simulink model "CVS_LVAD_2021a"  (R2021a)
settings: Solver=ode4  StartTime=0.0  StopTime=end_t  FixedStep=dt_step  RelTol=1e-3
values from neighbouring files (symbols this model uses):
  Cac = 13.7054    [SimMDL_Parameters.m]
  Cbc = 0.25    [SimMDL_Parameters.m]
  Cpa = 1/1.27    (= 0.787401574803)    [SimMDL_Parameters.m]
  Cpv = 1/0.247    (= 4.04858299595)    [SimMDL_Parameters.m]
  Csae = 1/3.02    (= 0.331125827815)    [SimMDL_Parameters.m]
  Csai = 1/7.76    (= 0.128865979381)    [SimMDL_Parameters.m]
  Csve = 1/0.0918    (= 10.8932461874)    [SimMDL_Parameters.m]
  Csvi = 1/0.0989    (= 10.111223458)    [SimMDL_Parameters.m]
  Da0 = 0    [SimMDL_Parameters.m]
  de_gain = 1.5    [SimMDL_Parameters.m]
  delay = 0.5*Tc    (= 0.230769230769)    [SimMDL_Parameters.m]
  deltastar = 0.5    [SimMDL_Parameters.m]
  DElv = 2*(Tc/0.833)    (= 1.10813556192)    [SimMDL_Parameters.m]
  DErv = 2*(Tc/0.833)    (= 1.10813556192)    [SimMDL_Parameters.m]
  Dm0 = 1    [SimMDL_Parameters.m]
  Dp0 = 0    [SimMDL_Parameters.m]
  DRsp = 3*(Tc/0.833)    (= 1.66220334288)    [SimMDL_Parameters.m]
  Dt0 = 1    [SimMDL_Parameters.m]
  dt_step = 1e-3    (= 0.001)    [SimMDL_Parameters.m]
  DTs = 3*(Tc/0.833)    (= 1.66220334288)    [SimMDL_Parameters.m]
  DTv = 0.5    [SimMDL_Parameters.m]
  e_gain = 2    [SimMDL_Parameters.m]
  Elamax = 1.99    [SimMDL_Parameters.m]
  Elamin = 0.733    [SimMDL_Parameters.m]
  Elvmax = 28.4    [SimMDL_Parameters.m]
  Elvmin = 0.550    (= 0.55)    [SimMDL_Parameters.m]
  Eramax = 0.63    [SimMDL_Parameters.m]
  Eramin = 0.317    [SimMDL_Parameters.m]
  Erv_max_sat = 1.2*Ervmax    (= 2.508)    [SimMDL_Parameters.m]
  Erv_max_thres = 0.8*Ervmax    (= 1.672)    [SimMDL_Parameters.m]
  Ervmax = 2.09    [SimMDL_Parameters.m]
  Ervmin = 0.348    [SimMDL_Parameters.m]
  Ga_Elv = 0.012    [SimMDL_Parameters.m]
  Ga_Erv = 0.012    [SimMDL_Parameters.m]
  Ga_Rsp = 0.1    [SimMDL_Parameters.m]
  GaTs = 0.015    [SimMDL_Parameters.m]
  GaTv = 0.028    [SimMDL_Parameters.m]
  Gp_Elv = 0    [SimMDL_Parameters.m]
  Gp_Erv = 0    [SimMDL_Parameters.m]
  Gp_Rsp = 0.33    [SimMDL_Parameters.m]
  GpTs = 0    [SimMDL_Parameters.m]
  GpTv = 0.25    [SimMDL_Parameters.m]
  k_Elv = (Elv_max_sat-Elv_max_thres)/(4*SElvo)    (= 2.84)    [SimMDL_Parameters.m]
  k_Erv = (Erv_max_sat-Erv_max_thres)/(4*SErvo)    (= 0.209)    [SimMDL_Parameters.m]
  k_Rsp = (Rsp_max-Rsp_min)/(4*SRspo)    (= 0.375)    [SimMDL_Parameters.m]
  Kn = max(Kn)    [SimMDL_Parameters.m]
  kT = (T_max-T_min)/(4*STo)    (= 0.035)    [SimMDL_Parameters.m]
  Li = 0.0402    [SimMDL_Parameters.m]
  Lo = 0.0426    [SimMDL_Parameters.m]
  Lsae = 0.0002    [SimMDL_Parameters.m]
  n = length(T)    [SimMDL_Parameters.m]
  pac0 = 0    [SimMDL_Parameters.m]
  pbc0 = 0    [SimMDL_Parameters.m]
  ppa0 = 8.5    [SimMDL_Parameters.m]
  ppv0 = 8    [SimMDL_Parameters.m]
  psae0 = 70    [SimMDL_Parameters.m]
  psai0 = 75    [SimMDL_Parameters.m]
  Psan = 75    [SimMDL_Parameters.m]
  psve0 = 8.7    [SimMDL_Parameters.m]
  psvi0 = 6    [SimMDL_Parameters.m]
  Pth = -3.25    [SimMDL_Parameters.m]
  qi0 = 0    [SimMDL_Parameters.m]
  qo0 = 0    [SimMDL_Parameters.m]
  qsae0 = 10    [SimMDL_Parameters.m]
  Rac = 0.0025    [SimMDL_Parameters.m]
  Ri = 0.4283    [SimMDL_Parameters.m]
  Rm = 0.006    [SimMDL_Parameters.m]
  Ro = 1.2841    [SimMDL_Parameters.m]
  Rpa = 0.006    [SimMDL_Parameters.m]
  Rpp = 0.220    (= 0.22)    [SimMDL_Parameters.m]
  Rpv = 0.006    [SimMDL_Parameters.m]
  Rsae = 0.120    (= 0.12)    [SimMDL_Parameters.m]
  Rsai = 0.016    [SimMDL_Parameters.m]
  Rsp = 2.00    (= 2)    [SimMDL_Parameters.m]
  Rsp_max = 3    [SimMDL_Parameters.m]
  Rsp_min = 1.5    [SimMDL_Parameters.m]
  Rsve = 0.18    [SimMDL_Parameters.m]
  Rsvi = 0.006    [SimMDL_Parameters.m]
  Rtv = 0.006    [SimMDL_Parameters.m]
  t_eject = (Tc*ts_VAD)/dt_step    (= 230.769230769)    [SimMDL_Parameters.m]
  T_max = 0.535    [SimMDL_Parameters.m]
  T_min = 0.395    [SimMDL_Parameters.m]
  Tas = 0.03+0.09*Tc    (= 0.0715384615385)    [SimMDL_Parameters.m]
  Tau_Elv = 1.5    [SimMDL_Parameters.m]
  Tau_Erv = 1.5    [SimMDL_Parameters.m]
  Tau_Rsp = 1.5    [SimMDL_Parameters.m]
  Tau_Ts = 1.8    [SimMDL_Parameters.m]
  Tau_Tv = 0.8    [SimMDL_Parameters.m]
  Tav = 0.01    [SimMDL_Parameters.m]
  Tc = 60/HR    (= 0.461538461538)    [SimMDL_Parameters.m]
  ts_VAD = 0.5    [SimMDL_Parameters.m]
  tune_alpha = x(5)    [SimMDL_Parameters.m]
  tune_gamma = x(3)    [SimMDL_Parameters.m]
  tune_lambda1 = x(1)    [SimMDL_Parameters.m]
  tune_lambda2 = x(2)    [SimMDL_Parameters.m]
  tune_nu = x(4)    [SimMDL_Parameters.m]
  Tvs = 0.16+0.20*Tc    (= 0.252307692308)    [SimMDL_Parameters.m]
  VAD_delay = ts_VAD    (= 0.5)    [SimMDL_Parameters.m]
  vla0 = 11.2524    [SimMDL_Parameters.m]
  Vlau = 1.0    (= 1)    [SimMDL_Parameters.m]
  Vln = 2.3    [SimMDL_Parameters.m]
  vlv0 = 15.6126    [SimMDL_Parameters.m]
  Vlvu = 2.0    (= 2)    [SimMDL_Parameters.m]
  vra0 = 22.36    [SimMDL_Parameters.m]
  Vrau = 1.5    [SimMDL_Parameters.m]
  vrv0 = 26.99    [SimMDL_Parameters.m]
  Vrvu = 3.0    (= 3)    [SimMDL_Parameters.m]
undefined symbols (not defined in the file or in its folder): D_E_max_lv, D_E_max_rv, D_R_svr, D_Ts, D_Tv, f_as_0, f_es_0, f_es_inf, f_es_min, f_ev_0, f_ev_inf, f_max, f_min, G_E_max_lv, G_E_max_rv, G_R_svr, G_Ts, G_Tv, HP_gain, HP_max, HP_min, HP_op, k_es, k_ev, ka, mPsai_op, mPsai_sat, mPsai_thres, passo, pn, Tau_E_max_lv, Tau_E_max_rv, Tau_p, Tau_R_svr, Tau_z
libraries: simulink x6, spsSampleandHoldLib x5, dspmathops x1
(part 1 of 2)
settings Model: SimulationMode=accelerator  Creator=RajarshiB  LastModifiedBy=RajarshiB

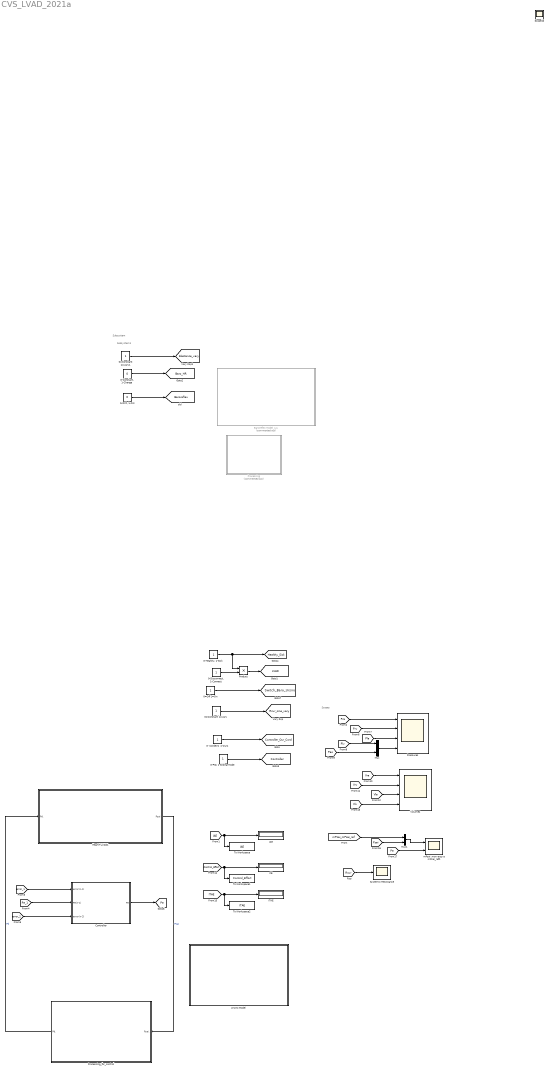
== system CVS_LVAD_2021a ==
  note: Subsystem
  note: Scopes
  note: Subsystem1
  0- Cordeiro  1-Ours : Constant
  "0-Constant, 1-Change" : Constant  Value=0
  "0-Disconnect, 1-Connect" : Constant
  "0-Healthy, 1-Sick" : Constant
  "0-OFF, 1-ON" : Constant  Value=0
  "0-PID, 1-Sliding-Mode" : Constant
  0=Constant 1=vary : Constant
  0=Constant 1=vary1 : Constant
  0=Off 1=On : Constant
  Baroreflex Model_Liu : Subsystem  Commented=on
  CE : Display
  Controller : Subsystem
  Heart+LVAD1 : Subsystem
  IAE : Display
  ITAE : Display
  Mux : Mux  Inputs=2
  Mux1 : Mux  Inputs=2
  Pressures : Scope  NumInputPorts=4
  Processing : Subsystem  Commented=on
  Processing_for_control : Subsystem
  Product : Product
  Systemic Resistance : Scope
  To Workspace : ToWorkspace  VariableName=IAE  SaveFormat=Timeseries  SampleTime=-1
  To Workspace1 : ToWorkspace  VariableName=Control_Effort  SaveFormat=Timeseries  SampleTime=-1
  To Workspace2 : ToWorkspace  VariableName=ITAE  SaveFormat=Timeseries  SampleTime=-1
  Ursino Model : Subsystem
  Volumes : Scope  NumInputPorts=4
  mPsai_mov-avg vs mPsai_ref1 : Scope  NumInputPorts=2
  Scope10 : Scope
  tag scope: Baro_HR=global, Baroreflex=global, Controller=global, Controller_Our_Cord=global, Elastance_vary=global, Healthy_Sick=global, LVAD=global, Pe=global, Rsvr_sine_vary=global, Switch_Baro_Ursino=global
  wires:
  Processing_for_control/1(Pd.) -> Heart+LVAD1/1(Pd.)  "Pd"
  Heart+LVAD1/1(Psai) -> Processing_for_control/1(Psai.)  "Psai"
  Controller/1(Pe) -> [Pe]
  [error_2] -> Controller/3(error(n-2))
  [Pe_1] -> Controller/2(Pe(n-1))
  [error_1] -> Controller/1(error(n-1))
  "0-Disconnect, 1-Connect"/1 -> Product/2
  [IAE] -> To Workspace/1, IAE/1
  "0-PID, 1-Sliding-Mode"/1 -> [Controller]
  "0-Healthy, 1-Sick"/1 -> Product/1, [Healthy_Sick]
  [Pao] -> Mux/2
  [Vrv] -> Volumes/2
  Mux/1 -> Pressures/4
  [Vlv] -> Volumes/4
  [Prv] -> Pressures/2
  [Pla] -> Pressures/3
  [Pra] -> Pressures/1
  [Plv] -> Mux/1
  [Vla] -> Volumes/3
  [Vra] -> Volumes/1
  [mPsai_mPsai_ref] -> Mux1/1
  [Control_Effort] -> To Workspace1/1, CE/1
  [ITAE] -> To Workspace2/1, ITAE/1
  [Psai] -> Mux1/2
  Mux1/1 -> mPsai_mov-avg vs mPsai_ref1/1
  [Pe] -> mPsai_mov-avg vs mPsai_ref1/2
  [Rsvr] -> Systemic Resistance/1
  0=Constant 1=vary/1 -> [Rsvr_sine_vary]
  0=Off 1=On/1 -> [Switch_Baro_Ursino]
  Product/1 -> [LVAD]
  0- Cordeiro  1-Ours/1 -> [Controller_Our_Cord]
  "0-OFF, 1-ON"/1 -> [Baroreflex]
  0=Constant 1=vary1/1 -> [Elastance_vary]
  "0-Constant, 1-Change"/1 -> [Baro_HR]

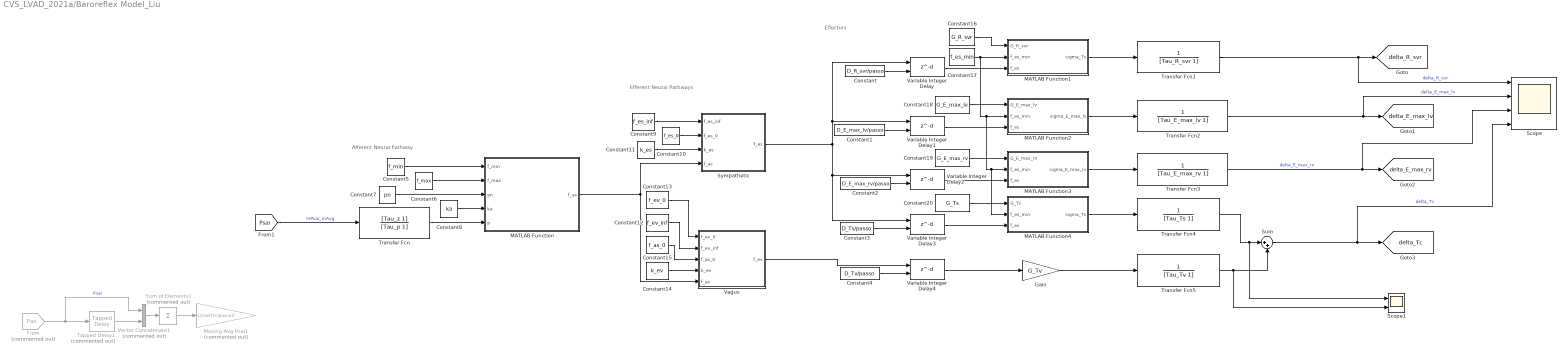
== system CVS_LVAD_2021a/Baroreflex Model_Liu ==
  note: Effectors
  note: Efferent Neural Pathways
  note: Afferent Neural Pathway
  Constant : Constant  Value=D_R_svr/passo
  Constant1 : Constant  Value=D_E_max_lv/passo
  Constant10 : Constant  Value=f_es_0
  Constant11 : Constant  Value=k_es
  Constant12 : Constant  Value=f_ev_inf
  Constant13 : Constant  Value=f_ev_0
  Constant14 : Constant  Value=k_ev
  Constant15 : Constant  Value=f_as_0
  Constant16 : Constant  Value=G_R_svr
  Constant17 : Constant  Value=f_es_min
  Constant18 : Constant  Value=G_E_max_lv
  Constant19 : Constant  Value=G_E_max_rv
  Constant2 : Constant  Value=D_E_max_rv/passo
  Constant20 : Constant  Value=G_Ts
  Constant3 : Constant  Value=D_Ts/passo
  Constant4 : Constant  Value=D_Tv/passo
  Constant5 : Constant  Value=f_min
  Constant6 : Constant  Value=f_max
  Constant7 : Constant  Value=pn
  Constant8 : Constant  Value=ka
  Constant9 : Constant  Value=f_es_inf
  From : From  Commented=on  GotoTag=Pao  TagVisibility=global
  Gain : Gain  Gain=G_Tv
  MATLAB Function : MATLAB Function  TreatAsAtomicUnit=on
  MATLAB Function1 : MATLAB Function  TreatAsAtomicUnit=on
  MATLAB Function2 : MATLAB Function  TreatAsAtomicUnit=on
  MATLAB Function3 : MATLAB Function  TreatAsAtomicUnit=on
  MATLAB Function4 : MATLAB Function  TreatAsAtomicUnit=on
  Moving-Avg Psai1 : Gain  Commented=on  Gain=1/(ceil(Tc/passo))
  Scope : Scope  NumInputPorts=4
  Scope1 : Scope  NumInputPorts=2
  Sum : Sum  Inputs=|++
  Sum of Elements1 : Sum  Commented=on  Inputs=+
  Sympathetic : MATLAB Function  TreatAsAtomicUnit=on
  Tapped Delay1 : simulink/Discrete/Tapped Delay  Commented=on  vinit=psai0  samptime=-1  NumDelays=ceil(Tc/passo)-1  DelayOrder=Oldest  includeCurrent=off
  Transfer Fcn : TransferFcn  Numerator=[Tau_z 1]  Denominator=[Tau_p 1]
  Transfer Fcn1 : TransferFcn  Denominator=[Tau_R_svr 1]
  Transfer Fcn2 : TransferFcn  Denominator=[Tau_E_max_lv 1]
  Transfer Fcn3 : TransferFcn  Denominator=[Tau_E_max_rv 1]
  Transfer Fcn4 : TransferFcn  Denominator=[Tau_Ts 1]
  Transfer Fcn5 : TransferFcn  Denominator=[Tau_Tv 1]
  Vagus : MATLAB Function  TreatAsAtomicUnit=on
  Variable Integer Delay{,1..4} (5 alike) : Delay  DelayLengthSource=Input port
      settings: InputPortMap=u0,p1
  Vector Concatenate1 : Concatenate  Commented=on
  tag scope: delta_E_max_lv=global, delta_E_max_rv=global, delta_R_svr=global, delta_Tc=global
  wires:
  Vagus/1(f_ev) -> Variable Integer Delay4/1
  Constant13/1 -> Vagus/1(f_ev_0)
  MATLAB Function/1(f_as) -> Vagus/5(f_as), Sympathetic/4(f_as)
  Constant18/1 -> MATLAB Function2/1(G_E_max_lv)
  Variable Integer Delay2/1 -> MATLAB Function3/3(f_es)
  Constant17/1 -> MATLAB Function1/2(f_es_min), MATLAB Function2/2(f_es_min), MATLAB Function4/2(f_es_min), MATLAB Function3/2(f_es_min)
  Constant10/1 -> Sympathetic/2(f_es_0)
  Variable Integer Delay3/1 -> MATLAB Function4/3(f_es)
  Constant4/1 -> Variable Integer Delay4/2
  Variable Integer Delay/1 -> MATLAB Function1/3(f_es)
  Transfer Fcn1/1 -> Scope/1, [delta_R_svr]  "delta_R_svr"
  Constant3/1 -> Variable Integer Delay3/2
  Transfer Fcn4/1 -> Scope1/1, Sum/1
  Constant11/1 -> Sympathetic/3(k_es)
  MATLAB Function2/1(sigma_E_max_lv) -> Transfer Fcn2/1
  Sympathetic/1(f_es) -> Variable Integer Delay3/1, Variable Integer Delay2/1, Variable Integer Delay1/1, Variable Integer Delay/1
  Constant5/1 -> MATLAB Function/1(f_min)
  Constant2/1 -> Variable Integer Delay2/2
  Constant12/1 -> Vagus/2(f_ev_inf)
  Variable Integer Delay4/1 -> Gain/1
  MATLAB Function1/1(sigma_Ts) -> Transfer Fcn1/1
  Constant1/1 -> Variable Integer Delay1/2
  Constant14/1 -> Vagus/4(k_ev)
  Constant15/1 -> Vagus/3(f_as_0)
  Constant16/1 -> MATLAB Function1/1(G_R_svr)
  Transfer Fcn/1 -> MATLAB Function/5(p)
  Transfer Fcn3/1 -> Scope/3, [delta_E_max_rv]  "delta_E_max_rv"
  Constant8/1 -> MATLAB Function/4(ka)
  Sum/1 -> Scope/4, [delta_Tc]  "delta_Tc"
  Transfer Fcn2/1 -> Scope/2, [delta_E_max_lv]  "delta_E_max_lv"
  Constant9/1 -> Sympathetic/1(f_es_inf)
  Gain/1 -> Transfer Fcn5/1
  Constant6/1 -> MATLAB Function/2(f_max)
  Constant20/1 -> MATLAB Function4/1(G_Ts)
  Constant/1 -> Variable Integer Delay/2
  Constant7/1 -> MATLAB Function/3(pn)
  Variable Integer Delay1/1 -> MATLAB Function2/3(f_es)
  Transfer Fcn5/1 -> Scope1/2, Sum/2
  MATLAB Function4/1(sigma_Ts) -> Transfer Fcn4/1
  MATLAB Function3/1(sigma_E_max_rv) -> Transfer Fcn3/1
  Constant19/1 -> MATLAB Function3/1(G_E_max_rv)
  Tapped Delay1/1 -> Vector Concatenate1/2
  Vector Concatenate1/1 -> Sum of Elements1/1
  Sum of Elements1/1 -> Moving-Avg Psai1/1
  From/1 -> Vector Concatenate1/1, Tapped Delay1/1  "Psai"
  [Psai] -> Transfer Fcn/1  "mPsai_mAvg"

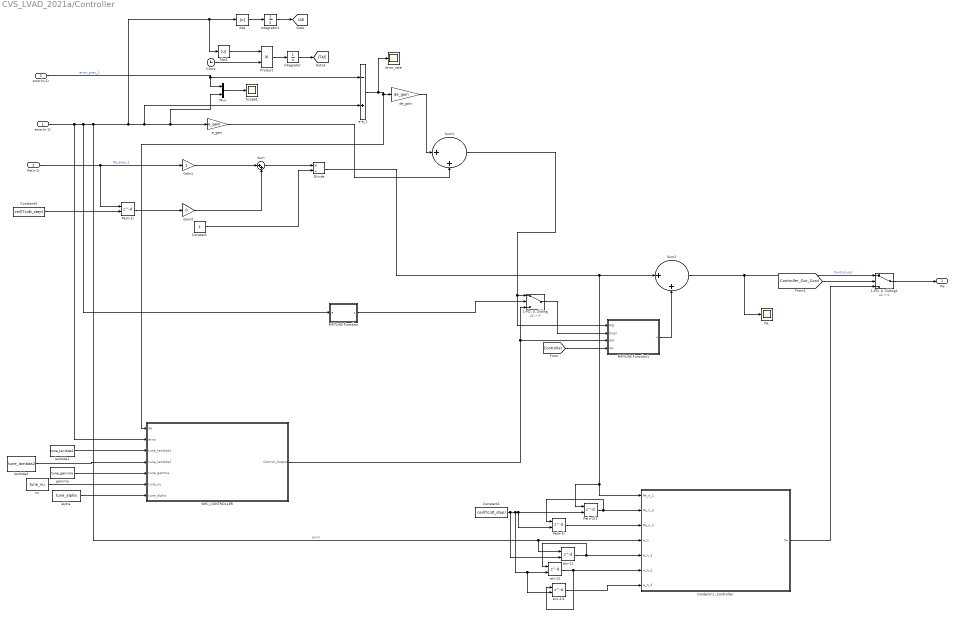
== system CVS_LVAD_2021a/Controller ==
  error(n-1) : Inport
  Pe(n-1) : Inport  Port=2
  error(n-2) : Inport  Port=3
  "1-PD, 0, Sliding" : Switch  Criteria=u2 > Threshold
  "1-PD, 0, Sliding1" : Switch  Criteria=u2 > Threshold
  Abs : Abs
  Abs1 : Abs
  Clock : Clock
  Constant : Constant
  Constant1 : Constant  Value=ceil(Tc/dt_step)
  Constant3 : Constant  Value=ceil(Tc/dt_step)
  Cordeiro's _Controller : MATLAB Function  TreatAsAtomicUnit=on
  Divide : Product  Inputs=*/
  Gain1 : Gain
  Gain3 : Gain  Gain=0
  Integrator : Integrator
  Integrator1 : Integrator
  MATLAB Function : MATLAB Function  TreatAsAtomicUnit=on
  MATLAB Function1 : MATLAB Function  TreatAsAtomicUnit=on
  Mux : Mux  Inputs=2
  Pe(n-2) : Delay  DelayLengthSource=Input port  InitialCondition=120
      settings: InputPortMap=u0,p1
  Pe(n-2)1 : Delay  DelayLengthSource=Input port  InitialCondition=120
      settings: InputPortMap=u0,p1
  Pe(n-3) : Delay  DelayLengthSource=Input port  InitialCondition=120
      settings: InputPortMap=u0,p1
  Pe. : Scope
  Product : Product
  "SMC_CONTROLLER " : Subsystem
  Scope1 : Scope
  Sum : Sum  Inputs=|++
  Sum1 : Sum  Inputs=|++
  Sum2 : Sum  Inputs=|++
  alpha : Constant  Value=tune_alpha
  de_gain : Gain  Gain=de_gain
  e(n-1) : Delay  DelayLengthSource=Input port  InitialCondition=120
      settings: InputPortMap=u0,p1
  e(n-2) : Delay  DelayLengthSource=Input port  InitialCondition=120
      settings: InputPortMap=u0,p1
  e(n-2)1 : Delay  DelayLengthSource=Input port  InitialCondition=120
      settings: InputPortMap=u0,p1
  e-e_1 : Sum  Inputs=-+
  e_gain : Gain  Gain=e_gain
  error_rate : Scope
  gamma : Constant  Value=tune_gamma
  lambda1 : Constant  Value=tune_lambda1
  lambda2 : Constant  Value=tune_lambda2
  nu : Constant  Value=tune_nu
  Pe : Outport
  tag scope: IAE=global, ITAE=global
  wires:
  Pe(n-1)/1 -> Gain1/1, Pe(n-2)/1  "Pe_prev_1"
  Gain1/1 -> Sum/1
  Mux/1 -> Scope1/1
  error(n-2)/1 -> e-e_1/1, Mux/1  "error_prev_1"
  e-e_1/1 -> error_rate/1, "SMC_CONTROLLER "/1(de), de_gain/1
  de_gain/1 -> Sum1/1
  Abs/1 -> Integrator1/1
  Integrator1/1 -> [IAE]
  Pe(n-2)/1 -> Gain3/1
  Gain3/1 -> Sum/2
  Sum/1 -> Divide/1
  Constant/1 -> Divide/2
  e_gain/1 -> Sum1/2
  Divide/1 -> Sum2/1, Pe(n-2)1/1, Cordeiro's _Controller/1(Pe_n_1)
  Constant3/1 -> Pe(n-2)/2
  Sum2/1 -> Pe./1, "1-PD, 0, Sliding1"/1  "Control_out"
  Sum1/1 -> MATLAB Function1/1(PID), "1-PD, 0, Sliding"/1
  "SMC_CONTROLLER "/1(Control_Output) -> "1-PD, 0, Sliding"/3, MATLAB Function1/3(SM)
  MATLAB Function/1(s) -> "1-PD, 0, Sliding"/2
  "1-PD, 0, Sliding"/1 -> MATLAB Function1/2(Dual)
  [Controller] -> MATLAB Function1/4(sw)
  MATLAB Function1/1(u) -> Sum2/2
  Abs1/1 -> Product/1
  Clock/1 -> Product/2
  Product/1 -> Integrator/1
  Integrator/1 -> [ITAE]
  lambda1/1 -> "SMC_CONTROLLER "/3(tune_lambda1)
  lambda2/1 -> "SMC_CONTROLLER "/4(tune_lambda2)
  gamma/1 -> "SMC_CONTROLLER "/5(tune_gamma)
  nu/1 -> "SMC_CONTROLLER "/6(tune_nu)
  alpha/1 -> "SMC_CONTROLLER "/7(tune_alpha)
  Pe(n-2)1/1 -> Pe(n-3)/1, Cordeiro's _Controller/2(Pe_n_2)
  Pe(n-3)/1 -> Cordeiro's _Controller/3(Pe_n_3)
  e(n-1)/1 -> e(n-2)/1, Cordeiro's _Controller/5(e_n_1)
  error(n-1)/1 -> "SMC_CONTROLLER "/2(error), MATLAB Function/1(e), e(n-1)/1, Cordeiro's _Controller/4(e_n), Abs/1, Abs1/1, e-e_1/2, Mux/2, e_gain/1  "error"
  e(n-2)1/1 -> Cordeiro's _Controller/7(e_n_3)
  e(n-2)/1 -> e(n-2)1/1, Cordeiro's _Controller/6(e_n_2)
  Constant1/1 -> e(n-1)/2, e(n-2)1/2, e(n-2)/2, Pe(n-3)/2, Pe(n-2)1/2
  "1-PD, 0, Sliding1"/1 -> Pe/1
  Cordeiro's _Controller/1(Pe) -> "1-PD, 0, Sliding1"/3
  [Controller_Our_Cord] -> "1-PD, 0, Sliding1"/2

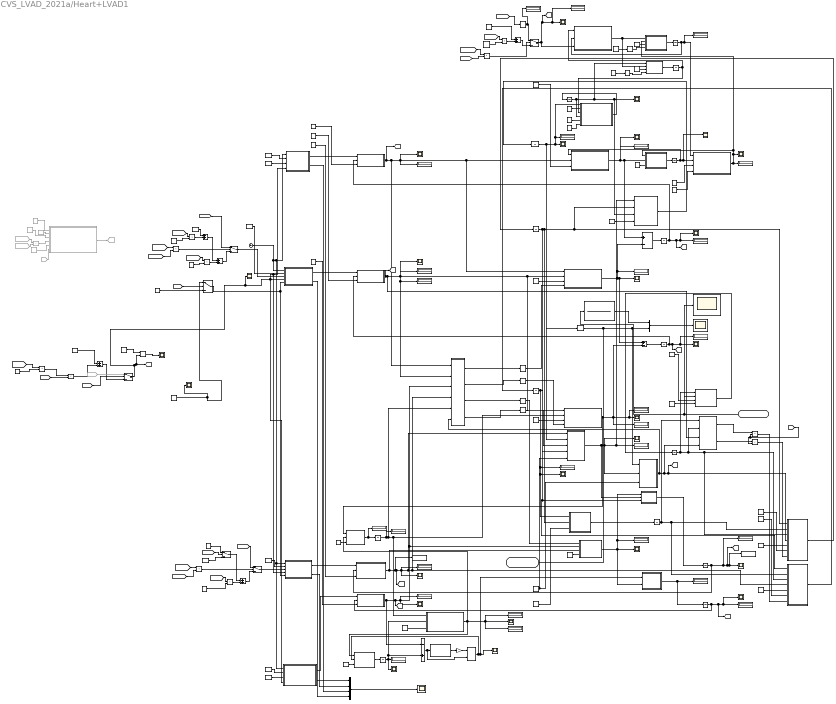
== system CVS_LVAD_2021a/Heart+LVAD1 ==
  note: Subsystem
  note: Subsystem7
  note: qla
  note: Subsystem8
  note: Subsystem1
  note: Subsystem6
  note: Subsystem5
  note: Subsystem3
  note: Subsystem4
  note: Subsystem2
  Pd. : Inport
  Add{,1..4} (5 alike) : Sum
  Clock2 : Clock
  Constant : Constant  Value=Rsai
  Constant1 : Constant  Value=Rsp
  Constant10 : Constant  Value=Cac
  Constant11 : Constant  Value=Ro
  Constant12 : Constant  Value=Lo
  Constant13 : Constant  Value=Csai
  Constant14 : Constant  Value=Csve
  Constant15 : Constant  Value=Csvi
  Constant16 : Constant  Value=Cpa
  Constant17 : Constant  Value=Rsae
  Constant18 : Constant  Value=Lsae
  Constant19 : Constant  Value=Pth
  Constant2 : Constant  Value=Rpa
  Constant20 : Constant  Value=Cpv
  Constant21 : Constant  Value=Rm
  Constant22 : Constant  Value=Kn
  Constant23 : Constant  Commented=on  Value=n
  Constant24 : Constant  Commented=on  Value=Tas
  Constant25 : Constant  Commented=on  Value=Tvs
  Constant26 : Constant  Commented=on  Value=Tav
  Constant27 : Constant  Value=60
  Constant28 : Constant  Value=9
  Constant{29,31,33,35,37} (5 alike) : Constant  Value=0
  Constant3 : Constant  Value=Pth
  Constant30 : Constant  Value=Tc
  Constant36 : Constant  Value=Kn
  Constant4 : Constant  Value=Rpp
  Constant5 : Constant  Value=Rsvi
  Constant6 : Constant  Value=Ri
  Constant7 : Constant  Value=Li
  Constant8 : Constant  Value=Cbc
  Constant9 : Constant  Value=Rac
  Csae : Constant  Value=Csae
  Da0 : Delay  DelayLength=1  InitialCondition=Da0
  Delay : Delay  DelayLength=1  InitialCondition=psai0
  Delay1 : Delay  DelayLength=1  InitialCondition=2
  Derivative : Derivative
  Derivative1 : Derivative
  Display{,1..17} (18 alike) : Display
  Divide : Product  Inputs=*/
  Dm0 : Delay  DelayLength=1  InitialCondition=Dm0
  Dp0 : Delay  DelayLength=1  InitialCondition=Dp0
  Dt0 : Delay  DelayLength=1  InitialCondition=Dt0
  Ela : MATLAB Function  TreatAsAtomicUnit=on
  Elamax : Constant  Value=Elamax
  Elamin : Constant  Value=Elamin
  Elv : MATLAB Function  TreatAsAtomicUnit=on
  Elvmax : Constant  Value=Elvmax
  Elvmin : Constant  Value=Elvmin
  Era : MATLAB Function  TreatAsAtomicUnit=on
  Eramax : Constant  Value=Eramax
  Eramin : Constant  Value=Eramin
  Erv : MATLAB Function  TreatAsAtomicUnit=on
  Ervmax : Constant  Value=Ervmax
  Ervmin : Constant  Value=Ervmin
  From12 : From  Commented=on  GotoTag=iteration  TagVisibility=global
  From21 : From  Commented=on  GotoTag=Baro_Tc
  From8 : From  Commented=on  GotoTag=Baroreflex  TagVisibility=global
  From9 : From  Commented=on  GotoTag=delta_Tc  TagVisibility=global
  Goto : Goto  Commented=on  GotoTag=Kn
  Heart_Valves : MATLAB Function  TreatAsAtomicUnit=on
  Klin : MATLAB Function  TreatAsAtomicUnit=on
  Kn_change : Scope
  Lvad_Valves : MATLAB Function  TreatAsAtomicUnit=on
  MATLAB Function : MATLAB Function  Commented=on  TreatAsAtomicUnit=on
  MiniMod : TransferFcn  Numerator=[1.033 10.74 6.623]  Denominator=[1 6.029 12.98 5.9]  ParameterTunability=Unconstrained
  Mux : Mux
  Mux1 : Mux  Inputs=2
  Pac_ : Integrator  InitialCondition=pac0
  Pao : MATLAB Function  TreatAsAtomicUnit=on
  Pbc_ : Integrator  InitialCondition=pbc0
  Pd : Scope
  Pla : MATLAB Function  TreatAsAtomicUnit=on
  Pla_Scope1 : Scope
  Plv : MATLAB Function  TreatAsAtomicUnit=on
  Plv_Scope2 : Scope
  Ppa : Integrator  InitialCondition=ppa0
  Ppa.. : Display
  Ppv : Integrator  InitialCondition=ppv0
  Ppv_Display : Display
  Pra = Ela*(Vra - Vrau) : MATLAB Function  TreatAsAtomicUnit=on
  Pra_Scope : Scope
  Product{,1..5,7,9..12} (11 alike) : Product
  Product6 : Product  Commented=on
  Prv = Erv*(Vrv - Vrvu) : MATLAB Function  TreatAsAtomicUnit=on
  Prv_Display : Display
  Prv_Scope1 : Scope
  Psae : Integrator  InitialCondition=psae0
  Psai_ : Integrator  InitialCondition=psai0
  Psai_Scope14 : Scope
  Psve : Integrator  InitialCondition=psve0
  Psvi : Integrator  InitialCondition=psvi0
  Rpv_ : Gain  Gain=Rpv
  Rsve : Constant  Value=Rsve
  Rtv : Constant  Value=Rtv
  Scope{,1..16,19} (18 alike) : Scope
  Subtract : Sum  Inputs=-+
  Switch{,1,3..5,7} (6 alike) : Switch  Criteria=u2 > Threshold
  To Workspace : ToWorkspace  VariableName=Plv  SaveFormat=Timeseries  SampleTime=-1
  To Workspace1 : ToWorkspace  VariableName=Vlv  SaveFormat=Timeseries  SampleTime=-1
  Vla : Display
  Vla. : Integrator  InitialCondition=vla0
  Vlau : Constant  Value=Vlau
  Vlv. : Integrator  InitialCondition=vlv0  UpperSaturationLimit=+1000  LowerSaturationLimit=-1000
  Vlvu : Constant  Value=Vlvu
  Vra : Integrator  InitialCondition=vra0
  Vrau : Constant  Value=Vrau
  Vrv : Integrator  InitialCondition=vrv0
  Vrvu : Constant  Value=Vrvu
  Vusae : Constant
  Vusve : Constant
  dPac/dt = (-1/(Rac*Cac))*Pac + (1/(Rac*Cac))*Pd : MATLAB Function  TreatAsAtomicUnit=on
  dPbc/dt = (1/Cbc)*qi - (1/Cbc)*qo : MATLAB Function  TreatAsAtomicUnit=on
  dPpa : Display
  dPpa/dt  = (qpa - qpp)/Cpa : MATLAB Function  TreatAsAtomicUnit=on
  dPpv/dt = (qpp - qla)/Cpv : MATLAB Function  TreatAsAtomicUnit=on
  dPsae/dt  = (qsae - qsp)/Csae : MATLAB Function  TreatAsAtomicUnit=on
  dPsai/dt  = (qsai + qo - qsae)/Csai : MATLAB Function  TreatAsAtomicUnit=on
  dPsve/dt  = (qsp - qsve)/Csve : MATLAB Function  TreatAsAtomicUnit=on
  dPsvi/dt  = (qsve - qra)/Csvi : MATLAB Function  TreatAsAtomicUnit=on
  dVla : Display
  dVla/dt  = qla - qmv : MATLAB Function  TreatAsAtomicUnit=on
  dVlv/dt  = qmv - qsai - qi : MATLAB Function  TreatAsAtomicUnit=on
  dVra/dt  = qra - qtv : Sum  Inputs=+-
  dVrv/dt  = qtv - qpa : Sum  Inputs=+-
  dqi/dt = -(Ri/Li)*qi - Di*(1/Li)*(Pbc+Pac) + Di*(1/Li)*plv : MATLAB Function  TreatAsAtomicUnit=on
  dqo/dt = -(Ro/Lo)*qo + Do*(1/Lo)*(Pac+Pbc) - Do*(1/Lo)*pao : MATLAB Function  TreatAsAtomicUnit=on
  dqsae/dt = (psai + Pth - psae - Rsae*qsae)/Lsae : MATLAB Function  TreatAsAtomicUnit=on
  qi_ : Integrator  InitialCondition=qi0
  qla = (Ppv- Pla)/(klin*Rpv) : Product  Inputs=/*
  qmv : Display
  qmv  = Dm*(Pla -  Plv)/Rmv : MATLAB Function  TreatAsAtomicUnit=on
  qo_ : Integrator  InitialCondition=qo0
  qpa : MATLAB Function  TreatAsAtomicUnit=on
  qpa_Display : Display
  qpp : MATLAB Function  TreatAsAtomicUnit=on
  qpp_Display : Display
  qra : MATLAB Function  TreatAsAtomicUnit=on
  qra_Scope1 : Scope
  qsae_ : Integrator  InitialCondition=qsae0  UpperSaturationLimit=1000  LowerSaturationLimit=-1000
  qsai : MATLAB Function  TreatAsAtomicUnit=on
  qsp : MATLAB Function  TreatAsAtomicUnit=on
  qsve : MATLAB Function  TreatAsAtomicUnit=on
  qtv : MATLAB Function  TreatAsAtomicUnit=on
  qtv_Scope1 : Scope
  qtv_Scope2 : Scope
  Psai : Outport
  tag scope: Pao=global, Pla=global, Plv=global, Pra=global, Prv=global, Rsvr=global, Tc=global, Vla=global, Vlv=global, Vra=global, Vrv=global
  wires:
  MiniMod/1 -> Mux1/1
  Constant11/1 -> dqo/dt = -(Ro/Lo)*qo + Do*(1/Lo)*(Pac+Pbc) - Do*(1/Lo)*pao/5(Ro)
  Constant12/1 -> dqo/dt = -(Ro/Lo)*qo + Do*(1/Lo)*(Pac+Pbc) - Do*(1/Lo)*pao/6(Lo)
  dPac/dt = (-1/(Rac*Cac))*Pac + (1/(Rac*Cac))*Pd/1(dPac) -> Pac_/1
  dqi/dt = -(Ri/Li)*qi - Di*(1/Li)*(Pbc+Pac) + Di*(1/Li)*plv/1(dqi) -> qi_/1
  Vrvu/1 -> Prv = Erv*(Vrv - Vrvu)/3(Vrvu)
  Lvad_Valves/1(Di) -> Product/1
  Constant3/1 -> qsve/3(Pth)
  Heart_Valves/1(Dt) -> Dt0/1
  Constant13/1 -> dPsai/dt  = (qsai + qo - qsae)/Csai/4(Csai)
  Prv = Erv*(Vrv - Vrvu)/1(Prv) -> [Prv], Display1/1, Heart_Valves/2(Prv), qpa/1(Prv), qtv/2(Prv), Prv_Display/1, Prv_Scope1/1, Lvad_Valves/3(Plv)
  Elamin/1 -> Ela/2(Elamin)
  Mux/1 -> Scope2/1
  Era/2(avt) -> Mux/3
  Clock2/1 -> Ela/1(Time), Elv/1(Time), Era/1(Time), Erv/1(Time)
  Constant2/1 -> qpa/3(Rpa)
  dPsve/dt  = (qsp - qsve)/Csve/1(Psve) -> Psve/1
  Product1/1 -> dqo/dt = -(Ro/Lo)*qo + Do*(1/Lo)*(Pac+Pbc) - Do*(1/Lo)*pao/7(Do)
  dPpa/dt  = (qpa - qpp)/Cpa/1(dPpa) -> dPpa/1, Ppa/1
  Vlau/1 -> Pla/3(Vlau)
  Heart_Valves/3(Dm) -> Dm0/1
  Rsve/1 -> qsve/4(Rsve)
  Constant14/1 -> dPsve/dt  = (qsp - qsve)/Csve/3(Csve)
  Eramin/1 -> Era/2(Eramin)
  dqsae/dt = (psai + Pth - psae - Rsae*qsae)/Lsae/1(dqsae) -> qsae_/1
  Elv/2(avt) -> Mux/2
  Constant4/1 -> qpp/3(Rpp)
  Ela/1(Ela) -> Pla/1(Ela)
  Erv/1(Erv) -> Prv = Erv*(Vrv - Vrvu)/1(Erv)
  Rtv/1 -> qtv/3(Rtv)
  Heart_Valves/2(Dp) -> Dp0/1
  dPpv/dt = (qpp - qla)/Cpv/1(dPpv) -> Ppv/1
  Heart_Valves/4(Da) -> Da0/1
  Eramax/1 -> Era/3(Eramax)
  Lvad_Valves/2(Do) -> Product1/1
  Dp0/1 -> qpa/4(Dp)
  Ervmin/1 -> Erv/2(Ervmin)
  Delay/1 -> Mux1/2, Pao/1(Psai), Psai/1
  Constant9/1 -> dPac/dt = (-1/(Rac*Cac))*Pac + (1/(Rac*Cac))*Pd/3(Rac)
  Product/1 -> dqi/dt = -(Ri/Li)*qi - Di*(1/Li)*(Pbc+Pac) + Di*(1/Li)*plv/7(Di)
  Vlvu/1 -> Plv/3(Vlvu)
  Pd./1 -> dPac/dt = (-1/(Rac*Cac))*Pac + (1/(Rac*Cac))*Pd/2(Pd), MiniMod/1, Pd/1  "Pd"
  Elvmin/1 -> Elv/2(Elvmin)
  Vrau/1 -> Pra = Ela*(Vra - Vrau)/3(Vrau)
  Subtract/1 -> Klin/1(Ppv_Pla), qla = (Ppv- Pla)/(klin*Rpv)/2
  dPbc/dt = (1/Cbc)*qi - (1/Cbc)*qo/1(dPbc) -> Pbc_/1
  Switch/1 -> Elv/3(Elvmax)
  dPsai/dt  = (qsai + qo - qsae)/Csai/1(dPsai) -> Psai_/1
  Psae/1 -> dqsae/dt = (psai + Pth - psae - Rsae*qsae)/Lsae/3(Psae), qsp/1(Psae)
  dVlv/dt  = qmv - qsai - qi/1(dVlv) -> Vlv./1
  Dt0/1 -> qtv/4(Dt)
  Constant6/1 -> dqi/dt = -(Ri/Li)*qi - Di*(1/Li)*(Pbc+Pac) + Di*(1/Li)*plv/5(Ri)
  Era/1(Era) -> Pra = Ela*(Vra - Vrau)/1(Era)
  Switch5/1 -> Erv/3(Ervmax)
  Ela/2(avt) -> Mux/1
  Elv/1(Elv) -> Plv/1(Elv)
  Erv/2(avt) -> Mux/4
  Da0/1 -> qsai/3(Da)
  Mux1/1 -> Scope15/1
  qsve/1(qsve) -> dPsve/dt  = (qsp - qsve)/Csve/2(qsve), dPsvi/dt  = (qsve - qra)/Csvi/1(qsve), qtv_Scope2/1, Display6/1  "qsve"
  Switch7/1 -> Elv/4(Tc), Era/4(Tc), Erv/4(Tc), Ela/4(Tc), Scope10/1, Divide/2, [Tc]  "HR"
  Elamax/1 -> Ela/3(Elamax)
  Constant8/1 -> dPbc/dt = (1/Cbc)*qi - (1/Cbc)*qo/3(Cbc)
  Constant7/1 -> dqi/dt = -(Ri/Li)*qi - Di*(1/Li)*(Pbc+Pac) + Di*(1/Li)*plv/6(Li)
  Constant10/1 -> dPac/dt = (-1/(Rac*Cac))*Pac + (1/(Rac*Cac))*Pd/4(Cac)
  dqo/dt = -(Ro/Lo)*qo + Do*(1/Lo)*(Pac+Pbc) - Do*(1/Lo)*pao/1(dqo) -> qo_/1
  Constant5/1 -> qra/3(Rsvi)
  qo_/1 -> dPsai/dt  = (qsai + qo - qsae)/Csai/2(qo), dqo/dt = -(Ro/Lo)*qo + Do*(1/Lo)*(Pac+Pbc) - Do*(1/Lo)*pao/1(qo), dPbc/dt = (1/Cbc)*qi - (1/Cbc)*qo/2(qo), qsai/4(qo)  "qo"
  Pbc_/1 -> dqo/dt = -(Ro/Lo)*qo + Do*(1/Lo)*(Pac+Pbc) - Do*(1/Lo)*pao/2(Pbc), dqi/dt = -(Ri/Li)*qi - Di*(1/Li)*(Pbc+Pac) + Di*(1/Li)*plv/2(Pbc), Lvad_Valves/1(Pbc)
  qtv/1(qtv) -> dVrv/dt  = qtv - qpa/1, qtv_Scope1/1, dVra/dt  = qra - qtv/2, Display5/1  "qtv"
  qsai/1(qsai) -> Display13/1, dPsai/dt  = (qsai + qo - qsae)/Csai/1(qsai), Pao/2(qsai), Scope8/1, dVlv/dt  = qmv - qsai - qi/2(qsai)
  Pao/1(Pao_) -> [Pao], dqo/dt = -(Ro/Lo)*qo + Do*(1/Lo)*(Pac+Pbc) - Do*(1/Lo)*pao/4(Pao), Lvad_Valves/4(Pao), Heart_Valves/6(Pao)
  qi_/1 -> dPbc/dt = (1/Cbc)*qi - (1/Cbc)*qo/1(qi), Scope6/1, Display11/1, dqi/dt = -(Ri/Li)*qi - Di*(1/Li)*(Pbc+Pac) + Di*(1/Li)*plv/1(qi), dVlv/dt  = qmv - qsai - qi/3(qi)
  Constant/1 -> Pao/3(Rsai), qsai/5(Rsai)
  Vlv./1 -> Display10/1, [Vlv], To Workspace1/1, Scope5/1, Plv/2(Vlv)
  Constant15/1 -> dPsvi/dt  = (qsve - qra)/Csvi/3(Csvi)
  Psai_/1 -> dqsae/dt = (psai + Pth - psae - Rsae*qsae)/Lsae/1(Psai), Display14/1, Psai_Scope14/1, qsai/2(Psai), Delay/1  "Psai"
  qsp/1(qsp) -> dPsve/dt  = (qsp - qsve)/Csve/1(qsp), dPsae/dt  = (qsae - qsp)/Csae/2(qsp)  "qsp"
  Vla./1 -> [Vla], Scope13/1, Vla/1, Pla/2(Vla)
  Ppa/1 -> qpp/1(Ppa), qpa/2(Ppa), Heart_Valves/5(Ppa), Ppa../1
  Plv/1(Plv) -> To Workspace/1, [Plv], Heart_Valves/4(Plv), dqi/dt = -(Ri/Li)*qi - Di*(1/Li)*(Pbc+Pac) + Di*(1/Li)*plv/4(Plv), qsai/1(Plv), Plv_Scope2/1, Display2/1, qmv  = Dm*(Pla -  Plv)/Rmv/3(Plv)
  Pra = Ela*(Vra - Vrau)/1(Pra) -> [Pra], qtv/1(Pra), qra/2(Pra), Display/1, Pra_Scope/1, Heart_Valves/1(Pra)
  dVla/dt  = qla - qmv/1(dVla) -> dVla/1, Vla./1
  [LVAD] -> Product/2, Product1/2
  qra/1(qra) -> dVra/dt  = qra - qtv/1, dPsvi/dt  = (qsve - qra)/Csvi/2(qra), Display4/1, qra_Scope1/1
  Pla/1(Pla) -> [Pla], qmv  = Dm*(Pla -  Plv)/Rmv/2(Pla), Heart_Valves/3(Pla), Pla_Scope1/1, Display3/1, Subtract/1
  Switch3/1 -> [Rsvr], Display15/1, Scope14/1, qsp/3(Rsp)
  Pac_/1 -> dqo/dt = -(Ro/Lo)*qo + Do*(1/Lo)*(Pac+Pbc) - Do*(1/Lo)*pao/3(Pac), dqi/dt = -(Ri/Li)*qi - Di*(1/Li)*(Pbc+Pac) + Di*(1/Li)*plv/3(Pac), Lvad_Valves/2(Pac), dPac/dt = (-1/(Rac*Cac))*Pac + (1/(Rac*Cac))*Pd/1(Pac)
  qpa/1(qpa) -> Scope1/1, Display8/1, dVrv/dt  = qtv - qpa/2, qpa_Display/1, dPpa/dt  = (qpa - qpp)/Cpa/1(qpa)
  Vrv/1 -> [Vrv], Display9/1, Scope4/1, Prv = Erv*(Vrv - Vrvu)/2(Vrv)
  qpp/1(qpp) -> qpp_Display/1, Display12/1, Scope7/1, dPpv/dt = (qpp - qla)/Cpv/1(qpp), dPpa/dt  = (qpa - qpp)/Cpa/2(qpp)
  Constant16/1 -> dPpa/dt  = (qpa - qpp)/Cpa/3(Cpa)
  Constant20/1 -> dPpv/dt = (qpp - qla)/Cpv/3(Cpv)
  Ppv/1 -> Subtract/2, qpp/2(Ppv), Ppv_Display/1, Scope11/1
  Constant21/1 -> qmv  = Dm*(Pla -  Plv)/Rmv/4(Rmv)
  qmv  = Dm*(Pla -  Plv)/Rmv/1(qmv) -> dVlv/dt  = qmv - qsai - qi/1(qmv), qmv/1, Scope9/1, dVla/dt  = qla - qmv/2(qmv)
  dPsvi/dt  = (qsve - qra)/Csvi/1(dPsvi) -> Psvi/1
  Psvi/1 -> Scope16/1, qsve/2(Psvi), qra/1(Psvi)
  Klin/1(Klin) -> Rpv_/1
  Rpv_/1 -> qla = (Ppv- Pla)/(klin*Rpv)/1
  qla = (Ppv- Pla)/(klin*Rpv)/1 -> dVla/dt  = qla - qmv/1(qla), Scope12/1, dPpv/dt = (qpp - qla)/Cpv/2(qla)
  Psve/1 -> Display16/1, qsve/1(Psve), qsp/2(Psve)
  Csae/1 -> dPsae/dt  = (qsae - qsp)/Csae/3(Csae)
  dPsae/dt  = (qsae - qsp)/Csae/1(dPsae) -> Psae/1
  Constant17/1 -> dqsae/dt = (psai + Pth - psae - Rsae*qsae)/Lsae/5(Rsae)
  Constant19/1 -> dqsae/dt = (psai + Pth - psae - Rsae*qsae)/Lsae/2(Pth)
  Constant18/1 -> dqsae/dt = (psai + Pth - psae - Rsae*qsae)/Lsae/6(Lsae)
  qsae_/1 -> dPsai/dt  = (qsai + qo - qsae)/Csai/3(qsae), Scope/1, dPsae/dt  = (qsae - qsp)/Csae/1(qsae), dqsae/dt = (psai + Pth - psae - Rsae*qsae)/Lsae/4(qsae)  "qsae"
  dVrv/dt  = qtv - qpa/1 -> Vrv/1
  dVra/dt  = qra - qtv/1 -> Vra/1
  Vra/1 -> [Vra], Scope3/1, Display7/1, Pra = Ela*(Vra - Vrau)/2(Vra)  "Vra"
  Dm0/1 -> qmv  = Dm*(Pla -  Plv)/Rmv/1(Dm)
  [Baroreflex] -> Product2/1
  Constant29/1 -> Product2/2
  Product2/1 -> Add/2
  Ervmax/1 -> Add/1
  Product3/1 -> Add1/2
  Switch1/1 -> Add1/1
  Constant33/1 -> Product3/2
  [Baroreflex] -> Product3/1
  Product4/1 -> Add2/2
  Constant1/1 -> Add2/1
  Constant37/1 -> Product4/2
  [Baroreflex] -> Product4/1
  MATLAB Function/1(Kn) -> Goto/1
  From9/1 -> Product6/2
  From8/1 -> Product6/1
  Product6/1 -> MATLAB Function/4(Tc)
  Constant23/1 -> MATLAB Function/5(n)
  Constant24/1 -> MATLAB Function/1(Tas)
  Constant26/1 -> MATLAB Function/2(Tav)
  Constant25/1 -> MATLAB Function/3(Tvs)
  From12/1 -> MATLAB Function/6(iter)
  Constant28/1 -> Switch1/1
  [Healthy_Sick] -> Switch1/2
  Elvmax/1 -> Switch1/3
  Add4/1 -> Switch7/3  "Tc"
  [Baroreflex] -> Product9/1
  Constant31/1 -> Product9/2
  Constant30/1 -> Add4/1  "Tc0"
  Product9/1 -> Product5/1
  [Baro_HR] -> Switch4/2
  Constant36/1 -> Kn_change/1, Switch4/1  "Kn"
  Constant22/1 -> Switch4/3
  Switch4/1 -> Erv/5(Kn), Elv/5(Kn)  "Kn"
  From21/1 -> Switch7/1
  [Baro_HR] -> Switch7/2
  [Baro_HR] -> Product5/2
  Product5/1 -> Add4/2
  Constant27/1 -> Divide/1
  Divide/1 -> Scope19/1  "HR"
  Add2/1 -> Switch3/3
  Delay1/1 -> Display17/1, Switch3/1
  Product7/1 -> Switch3/2
  [Baro_Rsp] -> Delay1/1
  [Switch_Baro_Ursino] -> Product7/1
  [Rsvr_sine_vary] -> Product7/2
  Vusae/1 -> Derivative/1
  Derivative/1 -> dPsae/dt  = (qsae - qsp)/Csae/4(Vusae_dot)
  Vusve/1 -> Derivative1/1
  Derivative1/1 -> dPsve/dt  = (qsp - qsve)/Csve/4(Vusve_dot)
  Add1/1 -> Switch/3
  [Switch_Baro_Ursino] -> Product10/1
  [Elastance_vary] -> Product10/2
  Product10/1 -> Switch/2
  [Elv_baro_ursino] -> Switch/1
  Product11/1 -> Switch5/2
  Add3/1 -> Switch5/3
  Product12/1 -> Add3/2
  [Baroreflex] -> Product12/1
  Add/1 -> Add3/1
  Constant35/1 -> Product12/2
  [Elastance_vary] -> Product11/2
  [Switch_Baro_Ursino] -> Product11/1
  [Erv_baro_ursino] -> Switch5/1

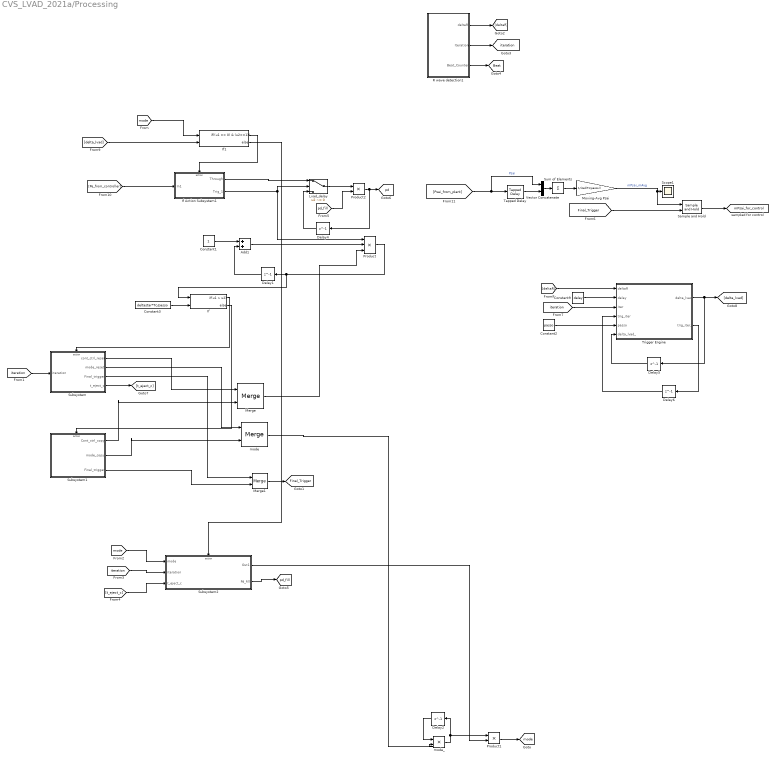
== system CVS_LVAD_2021a/Processing ==
  Add1 : Sum
  Constant1 : Constant
  Constant2 : Constant  Value=passo
  Constant3 : Constant  Value=deltastar*Tc/passo
  Constant9 : Constant  Value=delay
  Delay{1,4..6} (4 alike) : Delay  DelayLength=1
  Delay2 : Delay  DelayLength=1  InitialCondition=0
  If : If  NumInputs=2  IfExpression=u1 > u2
  If Action Subsystem1 : Subsystem  TreatAsAtomicUnit=on
  If1 : If  NumInputs=2  IfExpression=(u1 == 0) & (u2==1)
  Lvad_delay : Switch  Criteria=u2 ~= 0
  Merge : Merge
  Merge1 : Merge
  Moving-Avg Psai : Gain  Gain=1/(ceil(Tc/passo))
  Product : Product  Inputs=3
  Product1 : Product
  Product2 : Product
  R wave detection1 : Subsystem
  Sample and Hold : spsSampleandHoldLib/Sample and Hold  ic=0  Ts=passo
      settings: SourceProductBaseCode=PS
  Scope1 : Scope
  Subsystem : Subsystem
  Subsystem1 : Subsystem
  Subsystem2 : Subsystem
  Sum of Elements : Sum  Inputs=+
  Tapped Delay : simulink/Discrete/Tapped Delay  vinit=psai0  samptime=-1  NumDelays=ceil(Tc/passo)-1  DelayOrder=Oldest  includeCurrent=off
  Trigger Engine : MATLAB Function  TreatAsAtomicUnit=on
  Vector Concatenate : Concatenate
  mode : Merge
  mode_ : Product
  tag scope: Beat=global, Final_Trigger=global, iteration=global, mPsai_for_control=global, mode=global, pd=global, pd_fill=global
  wires:
  Sum of Elements/1 -> Moving-Avg Psai/1
  Constant9/1 -> Trigger Engine/2(delay)
  Lvad_delay/1 -> Product2/1
  [Psai_from_plant] -> Vector Concatenate/1, Tapped Delay/1  "Psai"
  Tapped Delay/1 -> Vector Concatenate/2
  Sample and Hold/1 -> [mPsai_for_control]
  Product/1 -> If/1, Delay1/1
  If Action Subsystem1/1(Through) -> Lvad_delay/1
  If/1 -> Subsystem/Action
  Trigger Engine/2(trig_iter_) -> Delay6/1
  Product2/1 -> Delay4/1, [pd]
  Product1/1 -> [mode]
  [Final_Trigger] -> Sample and Hold/2
  Add1/1 -> Product/2
  mode_/1 -> Delay2/1, Product1/1
  Vector Concatenate/1 -> Sum of Elements/1
  Constant2/1 -> Trigger Engine/5(passo)
  Delay1/1 -> Add1/2
  Trigger Engine/1(delta_lvad) -> Delay5/1, [delta_lvad]
  Moving-Avg Psai/1 -> Sample and Hold/1, Scope1/1  "mPsai_mAvg"
  Delay4/1 -> Lvad_delay/3
  If1/1 -> If Action Subsystem1/Action
  Delay2/1 -> mode_/1
  R wave detection1/3(Beat_Counter) -> [Beat]
  [Pe_from_controller] -> If Action Subsystem1/1(In1)
  [mode] -> If1/1
  Delay6/1 -> Trigger Engine/4(trig_iter)
  [delta_lvad] -> If1/2
  mode/1 -> mode_/2
  Constant3/1 -> If/2
  R wave detection1/1(deltaR) -> [deltaR]
  R wave detection1/2(Iteration) -> [iteration]
  Merge/1 -> Product/3
  Constant1/1 -> Add1/1
  [deltaR] -> Trigger Engine/1(deltaR)
  [pd_fill] -> Product2/2
  [iteration] -> Trigger Engine/3(iter)
  Delay5/1 -> Trigger Engine/6(delta_lvad_)
  Subsystem/1(cont_ctrl_reset) -> Merge/1
  Subsystem/2(mode_reset) -> mode/1
  Subsystem1/1(Cont_ctrl_copy) -> Merge/2
  Subsystem1/2(mode_copy) -> mode/2
  Subsystem/3(Final_trigger) -> Merge1/1
  Subsystem1/3(Final_trigger) -> Merge1/2
  Merge1/1 -> [Final_Trigger]
  Subsystem/4(t_eject_c) -> [t_eject_c]
  If/2 -> Subsystem1/Action
  [iteration] -> Subsystem/1(iteration)
  If Action Subsystem1/2(Trig_1) -> Product/1, Lvad_delay/2
  Subsystem2/1(Out1) -> Product1/2
  If1/2 -> Subsystem2/Action
  Subsystem2/2(Pd_fill) -> [pd_fill]
  [mode] -> Subsystem2/1(mode)
  [iteration] -> Subsystem2/2(iteration)
  [t_eject_c] -> Subsystem2/3(t_eject_c)

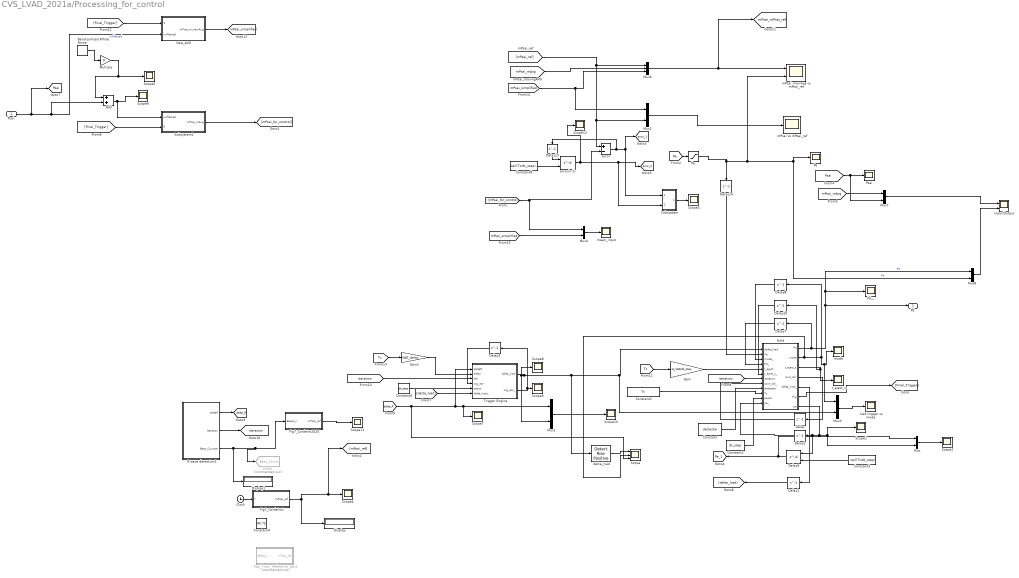
== system CVS_LVAD_2021a/Processing_for_control ==
  Psai. : Inport
  Add : Sum
  Band-Limited White Noise : simulink/Sources/Band-Limited White Noise  Cov=[0.0001]  Ts=dt_step  seed=[23341]
  Clock : Clock
  Constant : Constant  Value=deltastar
  Constant1 : Constant  Value=Tc
  Constant2 : Constant  Value=dt_step
  Constant3 : Constant  Value=ceil(Tc/dt_step)
  Constant4 : Constant  Value=80.75
  Constant6 : Constant  Value=dt_step
  Constant8 : Constant  Value=ceil(Tc/dt_step)-1  SampleTime=-1
  Delay : Delay  DelayLength=1  InitialCondition=0
  Delay1 : Delay  DelayLength=1  InitialCondition=0
  Delay10 : Delay  DelayLength=1  InitialCondition=t_eject
  Delay{3,7,13..14} (4 alike) : Delay  DelayLength=1
  Delay2 : Delay  DelayLength=1  InitialCondition=120
  Delay8 : Delay  DelayLength=1  InitialCondition=0
  Delay9 : Delay  DelayLengthSource=Input port  DelayLength=1  DelayLengthUpperLimit=10000  InitialCondition=120
      settings: InputPortMap=u0,p1
  Display : Display
  Display1 : Display
  Fig7_Cordeiro1 : MATLAB Function  TreatAsAtomicUnit=on
  Fig7_Cordeiro2020 : MATLAB Function  TreatAsAtomicUnit=on
  Gain : Gain  Gain=ts_VAD/dt_step
  Gain1 : Gain  Gain=VAD_delay
  Goto6 : Goto  Commented=on  GotoTag=Beat_Count  TagVisibility=global
  Hold : MATLAB Function  TreatAsAtomicUnit=on
  Input/Output : Scope  NumInputPorts=2
  Multiply : Gain  Gain=0
  Mux{,1..4,7..8} (7 alike) : Mux  Inputs=2
      Mux1 settings: DisplayOption=signals
  Mux6 : Mux  Inputs=3
  New_AVG : Subsystem
  Pd__ : Scope
  Pe : Scope
  Pe. : Saturate  UpperLimit=300  LowerLimit=-20
  Psai : Scope
  Psai_Train_Reference_gen1 : MATLAB Function  Commented=on  TreatAsAtomicUnit=on
  R wave detection1 : Subsystem
  Scope : Scope  NumInputPorts=3
  Scope{1..12} (12 alike) : Scope
  Subsystem : Subsystem
  Subsystem1 : Subsystem
  Trigger Engine : MATLAB Function  TreatAsAtomicUnit=on
  delta_lvad : simulink/Logic and Bit Operations/Detect Rise Positive  vinit=0  OutDataTypeStr=boolean
  error : Sum  Inputs=+-
  error(n-1). : Delay  DelayLengthSource=Input port  DelayLength=1  DelayLengthUpperLimit=10000  InitialCondition=0  SampleTime=dt_step
      settings: InputPortMap=u0,p1
  lvad trigger vs mode : Scope
  mPsai vs mPsai_ref : Scope
  mPsai_mov-avg vs mPsai_ref : Scope  NumInputPorts=2
  mean_input : Scope
  mode : Scope
  t_eject_c : Scope
  Pd. : Outport
  tag scope: Pe_1=global, Psai=global, delta_R=global, error_1=global, error_2=global, iteration=global, mPsai_mPsai_ref=global, mPsai_simplified=global
  wires:
  Delay10/1 -> Hold/6(t_eject_c_)
  Mux2/1 -> mPsai vs mPsai_ref/1
  Mux1/1 -> Scope10/1
  Delay7/1 -> Hold/4(Pd_)
  Delay8/1 -> Hold/3(mode_)
  Constant6/1 -> Trigger Engine/5(passo)
  Gain/1 -> Hold/5(t_eject)
  [mPsai_ref] -> error/1, Mux2/2, Mux6/1
  Gain1/1 -> Trigger Engine/2(delay)
  Mux3/1 -> lvad trigger vs mode/1
  Delay3/1 -> Trigger Engine/4(trig_iter)
  Hold/1(Pd) -> Mux8/1, Pd__/1, Pd./1, Delay7/1  "Pd"
  Pe./1 -> mPsai_mov-avg vs mPsai_ref/2, Mux8/2, Pe/1, Delay14/1  "Pe"
  Hold/3(t_eject_c) -> t_eject_c/1, Delay10/1
  Trigger Engine/2(trig_iter_) -> Delay3/1, Scope9/1
  [delta_R] -> Scope/3, Scope7/1, Mux1/1, Trigger Engine/1(deltaR)
  error/1 -> Delay13/1, [error_1], Subsystem/1(e(n))
  Hold/4(cont_ctrl) -> Delay/1
  Delay/1 -> Hold/8(cont_ctrl_)
  Constant/1 -> Hold/9(deltastar)
  Constant1/1 -> Hold/10(Tc)
  Constant2/1 -> Hold/11(passo)
  Hold/5(delta_lvad_) -> Delay1/1
  Hold/6(trig) -> [Final_Trigger]
  R wave detection1/3(Beat_Counter) -> Goto6/1, Fig7_Cordeiro2020/1(Beats_c), Display1/1
  Hold/7(pe) -> Scope1/1, Mux/2, Delay9/1, Delay2/1
  Delay2/1 -> Hold/12(pe_)
  Mux/1 -> Scope2/1
  Constant3/1 -> Delay9/2
  Delay9/1 -> Mux/1, [Pe_1]
  Constant8/1 -> error(n-1)./2
  error(n-1)./1 -> Scope12/1, Subsystem/2(e(n-1)), [error_2]
  Subsystem/1(de/dt) -> Scope3/1
  [mPsai_simplified] -> Mux4/2
  [Pe] -> Pe./1
  Delay13/1 -> error(n-1)./1
  Delay14/1 -> Hold/2(Pe)
  Mux7/1 -> Input/Output/1
  Mux8/1 -> Input/Output/2
  Fig7_Cordeiro2020/1(mPsai_ref) -> Scope11/1
  [mPsai_mAvg] -> Mux7/1
  [Psai] -> Mux7/2, Psai/1
  [mPsai_mAvg] -> Mux6/2
  Delay1/1 -> [delta_lvad]
  [delta_lvad] -> Trigger Engine/6(delta_lvad_)
  R wave detection1/1(deltaR) -> [delta_R]
  R wave detection1/2(Iteration) -> [iteration]
  [iteration] -> Hold/7(iteration)
  [iteration] -> Trigger Engine/3(iter)
  Mux6/1 -> [mPsai_mPsai_ref], mPsai_mov-avg vs mPsai_ref/1
  Psai./1 -> [Psai], Add/2, New_AVG/2(unfiltered)  "unfiltered"
  [mPsai_simplified] -> Mux2/1, Mux6/3
  Mux4/1 -> mean_input/1
  [mPsai_for_control] -> Mux4/1, error/2
  [Final_Trigger] -> Subsystem1/2(S)
  [Final_Trigger] -> New_AVG/1(S)
  New_AVG/1(mPsai_m_newAvg) -> [mPsai_simplified]
  [Tc] -> Gain/1
  [Tc] -> Gain1/1
  Trigger Engine/1(delta_lvad) -> delta_lvad/1, Hold/1(delta_lvad), Mux3/2, Scope8/1, Mux1/2
  delta_lvad/1 -> Scope/1
  Hold/2(mode) -> Scope/2, mode/1, Mux3/1, Delay8/1
  Clock/1 -> Fig7_Cordeiro1/1(t)
  Subsystem1/1(mPsai_mAvg) -> [mPsai_for_control]
  Add/1 -> Subsystem1/1(unfiltered), Scope6/1
  Multiply/1 -> Add/1, Scope5/1
  Band-Limited White Noise/1 -> Multiply/1
  Fig7_Cordeiro1/1(mPsai_ref) -> Display/1, Scope4/1, [mPsai_ref]

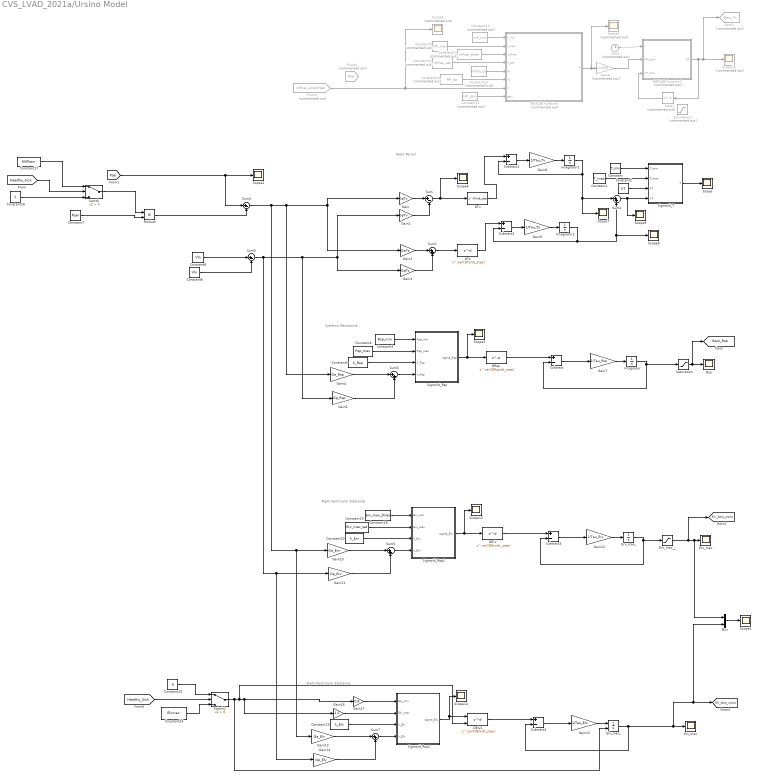
== system CVS_LVAD_2021a/Ursino Model ==
  note: Systemic Resistance
  note: Heart Period
  note: Right Ventricular Elastance
  note: Right Ventricular Elastance
  Clock : Clock  Commented=on
  Constant : Constant  Value=T_min
  Constant1 : Constant  Value=T_max
  Constant10 : Constant  Commented=on  Value=HP_min
  Constant11 : Constant  Commented=on  Value=mPsai_thres
  Constant12 : Constant  Commented=on  Value=mPsai_sat
  Constant13 : Constant  Commented=on  Value=mPsai_op
  Constant14 : Constant  Commented=on  Value=HP_op
  Constant15 : Constant  Commented=on  Value=HP_gain
  Constant16 : Constant
  Constant17 : Constant  Value=65/Psan
  Constant18 : Constant  Value=Erv_max_thres
  Constant19 : Constant  Value=Erv_max_sat
  Constant2 : Constant  Value=kT
  Constant20 : Constant  Value=k_Erv
  Constant23 : Constant  Value=k_Elv
  Constant24 : Constant  Value=Elvmax
  Constant25 : Constant  Value=9
  Constant3 : Constant  Value=Rsp_min
  Constant4 : Constant  Value=Rsp_max
  Constant5 : Constant  Value=k_Rsp
  Constant6 : Constant  Value=Vln
  Constant7 : Constant  Value=Psan
  Constant8 : Constant  Value=Vln
  Constant9 : Constant  Commented=on  Value=HP_max
  DElv1 : Delay  DelayLength=ceil(DElv/dt_step)  InitialConditionSource=Input port  InitialCondition=2
      settings: InputPortMap=u0,p4
  DErv : Delay  DelayLength=ceil(DErv/dt_step)  InitialCondition=2
  DRsp : Delay  DelayLength=ceil(DRsp/dt_step)  InitialCondition=2
  DTs : Delay  DelayLength=ceil(DTs/dt_step)  InitialCondition=(psai0-Psan)*GaTs
  DTv : Delay  DelayLength=DTv/dt_step  InitialCondition=(psai0-Psan)*GaTv
  Delay : Delay  Commented=on  DelayLength=1  InitialCondition=Tc
  Elv_max : Scope
  Elv_max_ : Integrator  InitialConditionSource=external  InitialCondition=28.33
  Erv_max : Scope
  Erv_max_ : Integrator  InitialCondition=Ervmax
  Erv_max__ : Saturate  UpperLimit=4  LowerLimit=1.5
  From3 : From  Commented=on  GotoTag=mPsai_simplified  TagVisibility=global
  From4 : From  Commented=on  GotoTag=Psai  TagVisibility=global
  Gain : Gain  Gain=GaTv
  Gain1 : Gain  Gain=GpTv
  Gain10 : Gain  Gain=Ga_Erv
  Gain11 : Gain  Gain=Gp_Erv
  Gain12 : Gain  Gain=1/Tau_Erv
  Gain13 : Gain  Gain=Ga_Elv
  Gain14 : Gain  Gain=Gp_Elv
  Gain15 : Gain  Gain=1/Tau_Elv
  Gain16 : Gain  Gain=1.2
  Gain17 : Gain  Gain=0.8
  Gain2 : Gain  Gain=GaTs
  Gain3 : Gain  Gain=GpTs
  Gain4 : Gain  Gain=Ga_Rsp
  Gain5 : Gain  Gain=Gp_Rsp
  Gain6 : Gain  Commented=on  Gain=1/1000
  Gain7 : Gain  Gain=1/Tau_Rsp
  Gain8 : Gain  Gain=1/Tau_Tv
  Gain9 : Gain  Gain=1/Tau_Ts
  Goto1 : Goto  Commented=on  GotoTag=Baro_Tc  TagVisibility=global
  Integrator : Integrator  InitialCondition=2
  Integrator1 : Integrator  InitialCondition=0.365
  Integrator2 : Integrator  InitialCondition=0.1
  MATLAB Function : MATLAB Function  Commented=on  TreatAsAtomicUnit=on
  MATLAB Function1 : MATLAB Function  Commented=on  TreatAsAtomicUnit=on
  Mux : Mux  Inputs=2
  Product : Product
  Rsp : Scope
  Saturation : Saturate  UpperLimit=Rsp_max  LowerLimit=Rsp_min
  Saturation1 : Saturate  Commented=on
  Scope{,1..4,7..9,12,14} (10 alike) : Scope
  Scope10 : Scope  Commented=on
  Scope5 : Scope  Commented=on
  Scope6 : Scope  Commented=on
  Sigmoid_Rsp : MATLAB Function  TreatAsAtomicUnit=on
  Sigmoid_Rsp1 : MATLAB Function  TreatAsAtomicUnit=on
  Sigmoid_Rsp2 : MATLAB Function  TreatAsAtomicUnit=on
  Sigmoid_T : MATLAB Function  TreatAsAtomicUnit=on
  Subtract{,1..4} (5 alike) : Sum  Inputs=+-
  Sum : Sum  Inputs=|+-
  Sum{1..3,6..7} (5 alike) : Sum  Inputs=|++
  Sum4 : Sum  Inputs=|+-
  Sum5 : Sum  Inputs=|+-
  Switch : Switch  Criteria=u2 > Threshold
  Switch1 : Switch  Criteria=u2 > Threshold
  tag scope: Baro_Rsp=global, Elv_baro_ursino=global, Erv_baro_ursino=global
  wires:
  Sigmoid_Rsp/1(sigma_Rsp) -> Scope3/1, DRsp/1
  Constant6/1 -> Sum5/2
  Constant5/1 -> Sigmoid_Rsp/3(k_Rsp)
  Constant2/1 -> Sigmoid_T/3(kT)
  Integrator2/1 -> Scope8/1, Sum2/2, Subtract2/2
  Gain3/1 -> Sum1/2
  Product/1 -> Sum4/2
  Sum2/1 -> Scope9/1, Sigmoid_T/4(xT)
  Sum3/1 -> Sigmoid_Rsp/4(x_Rsp)
  Constant/1 -> Sigmoid_T/1(T_min)
  Integrator/1 -> Subtract/2, Saturation/1
  DRsp/1 -> Subtract/1
  Constant3/1 -> Sigmoid_Rsp/1(Rsp_min)
  Gain2/1 -> Sum1/1
  Gain1/1 -> Sum/2
  Constant1/1 -> Sigmoid_T/2(T_max)
  [Psai] -> Sum4/1, Scope2/1
  Gain/1 -> Sum/1
  Constant8/1 -> Sum5/1
  Gain4/1 -> Sum3/1
  Gain5/1 -> Sum3/2
  Integrator1/1 -> Scope7/1, Sum2/1, Subtract1/2
  Constant4/1 -> Sigmoid_Rsp/2(Rsp_max)
  Saturation/1 -> [Baro_Rsp], Rsp/1
  Sum1/1 -> DTs/1
  Sum/1 -> DTv/1, Scope4/1
  Constant15/1 -> MATLAB Function/8(gain)
  Constant14/1 -> MATLAB Function/6(Y0)
  Constant13/1 -> MATLAB Function/5(X0)
  Constant11/1 -> MATLAB Function/3(X_thres)
  Constant12/1 -> MATLAB Function/4(X_sat)
  Constant9/1 -> MATLAB Function/2(Y_max)
  MATLAB Function/1(Y) -> Scope5/1, Gain6/1
  From3/1 -> Scope6/1, MATLAB Function/7(X)
  Constant10/1 -> MATLAB Function/1(Y_min)
  Sigmoid_T/1(T) -> Scope/1
  Subtract/1 -> Gain7/1
  Gain7/1 -> Integrator/1
  Gain8/1 -> Integrator1/1
  Subtract1/1 -> Gain8/1
  DTv/1 -> Subtract1/1
  Gain9/1 -> Integrator2/1
  Subtract2/1 -> Gain9/1
  DTs/1 -> Subtract2/1
  Clock/1 -> MATLAB Function1/1(t)
  Gain6/1 -> MATLAB Function1/2(HP_baro)
  MATLAB Function1/1(HP) -> Goto1/1, Scope10/1, Delay/1
  Delay/1 -> MATLAB Function1/3(HP_Prev)
  Switch/1 -> Product/1
  Constant7/1 -> Product/2
  Constant16/1 -> Switch/3
  Constant17/1 -> Switch/1
  [Healthy_Sick] -> Switch/2
  Constant19/1 -> Sigmoid_Rsp1/2(Erv_max)
  Gain12/1 -> Erv_max_/1
  Sigmoid_Rsp1/1(sigma_Erv) -> Scope12/1, DErv/1
  Erv_max_/1 -> Subtract3/2, Erv_max__/1
  Constant18/1 -> Sigmoid_Rsp1/1(Erv_min)
  Erv_max__/1 -> [Erv_baro_ursino], Mux/1, Erv_max/1
  Gain11/1 -> Sum6/2
  Sum6/1 -> Sigmoid_Rsp1/4(x_Erv)
  Gain10/1 -> Sum6/1
  Constant20/1 -> Sigmoid_Rsp1/3(k_Erv)
  DErv/1 -> Subtract3/1
  Subtract3/1 -> Gain12/1
  Subtract4/1 -> Gain15/1
  Sum4/1 -> Gain13/1, Gain10/1, Gain4/1, Gain2/1, Gain/1
  Constant23/1 -> Sigmoid_Rsp2/3(k_Elv)
  DElv1/1 -> Subtract4/1
  Gain13/1 -> Sum7/1
  Gain14/1 -> Sum7/2
  Sum7/1 -> Sigmoid_Rsp2/4(x_Elv)
  Sum5/1 -> Gain14/1, Gain11/1, Gain5/1, Gain1/1, Gain3/1
  Gain17/1 -> Sigmoid_Rsp2/1(Elv_min)
  Sigmoid_Rsp2/1(sigma_Elv) -> Scope14/1, DElv1/1
  Elv_max_/1 -> Mux/2, [Elv_baro_ursino], Elv_max/1, Subtract4/2
  Gain16/1 -> Sigmoid_Rsp2/2(Elv_max)
  Gain15/1 -> Elv_max_/1
  Constant24/1 -> Switch1/3
  Constant25/1 -> Switch1/1
  Switch1/1 -> Elv_max_/2, DElv1/2, Gain16/1, Gain17/1
  [Healthy_Sick] -> Switch1/2
  Mux/1 -> Scope1/1

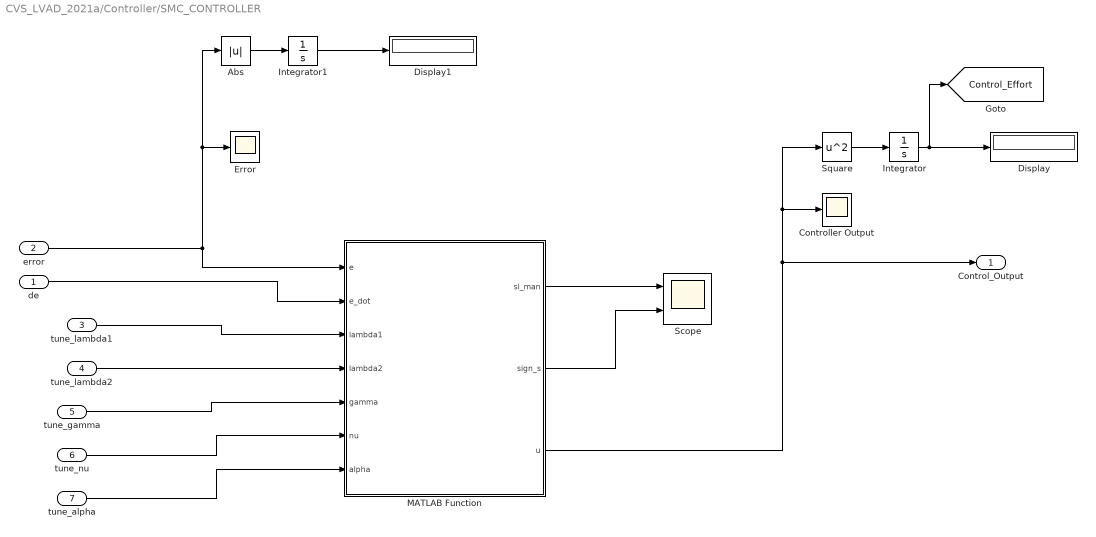
== system CVS_LVAD_2021a/Controller/SMC_CONTROLLER  ==
  de : Inport
  error : Inport  Port=2
  tune_lambda1 : Inport  Port=3
  tune_lambda2 : Inport  Port=4
  tune_gamma : Inport  Port=5
  tune_nu : Inport  Port=6
  tune_alpha : Inport  Port=7
  Abs : Abs
  Controller Output : Scope
  Display : Display
  Display1 : Display
  Error : Scope
  Integrator : Integrator
  Integrator1 : Integrator
  MATLAB Function : MATLAB Function  TreatAsAtomicUnit=on
  Scope : Scope  NumInputPorts=2
  Square : Math  Operator=square  SaturateOnIntegerOverflow=on
  Control_Output : Outport
  tag scope: Control_Effort=global
  wires:
  error/1 -> MATLAB Function/1(e), Abs/1, Error/1
  MATLAB Function/3(u) -> Controller Output/1, Square/1, Control_Output/1
  Integrator/1 -> [Control_Effort], Display/1
  Square/1 -> Integrator/1
  Integrator1/1 -> Display1/1
  Abs/1 -> Integrator1/1
  de/1 -> MATLAB Function/2(e_dot)
  tune_lambda1/1 -> MATLAB Function/3(lambda1)
  tune_lambda2/1 -> MATLAB Function/4(lambda2)
  tune_gamma/1 -> MATLAB Function/5(gamma)
  tune_nu/1 -> MATLAB Function/6(nu)
  tune_alpha/1 -> MATLAB Function/7(alpha)
  MATLAB Function/1(sl_man) -> Scope/1
  MATLAB Function/2(sign_s) -> Scope/2

== system CVS_LVAD_2021a/Processing/If Action Subsystem1 ==
  In1 : Inport
  Action Port : ActionPort  ActionPortLabel=if((u1 == 0) & (u2==1))
  Constant : Constant
  Through : Outport
  Trig_1 : Outport  Port=2
  wires:
  In1/1 -> Through/1
  Constant/1 -> Trig_1/1

== system CVS_LVAD_2021a/Processing/R wave detection1 ==
  Clock : Clock
  Constant1 : Constant  Value=dt_step
  Delay : Delay  DelayLength=1
  Delay1 : Delay  DelayLength=1  InitialCondition=0
  Display : Display
  MATLAB Function1 : MATLAB Function  TreatAsAtomicUnit=on
  deltaR : Outport
  Iteration : Outport  Port=2
  Beat_Counter : Outport  Port=3
  wires:
  MATLAB Function1/2(aux) -> Delay/1
  MATLAB Function1/1(iter) -> Display/1, Iteration/1
  Clock/1 -> MATLAB Function1/1(t)
  [HR] -> MATLAB Function1/2(HR)
  Constant1/1 -> MATLAB Function1/4(passo)
  MATLAB Function1/3(deltaR) -> deltaR/1
  Delay/1 -> MATLAB Function1/3(aux_)
  MATLAB Function1/4(Beat_Counter) -> Beat_Counter/1, Delay1/1
  Delay1/1 -> MATLAB Function1/5(Beat_Counter_)
